simulink model "analog_digital_comp"  (R2018a)
settings: Solver=VariableStepAuto  StartTime=0.0  StopTime=5  RelTol=1e-3
values from neighbouring files (symbols this model uses):
  Fs = 2*f    (= 88200)    [Project_Script.m]
libraries: dspvision x4, commchan3 x2, commutil2 x2, dspquant2 x2, dsparch4 x1, dspsigattribs x1, dspstat3 x1
settings Model: Creator=Mehdi Raza Khorasani  LastModifiedBy=Ali
settings DataIOCC: ReturnWorkspaceOutputs=on
settings SFSimCC: SimUseLocalCustomCode=on
settings RTWCC: RTWUseLocalCustomCode=on

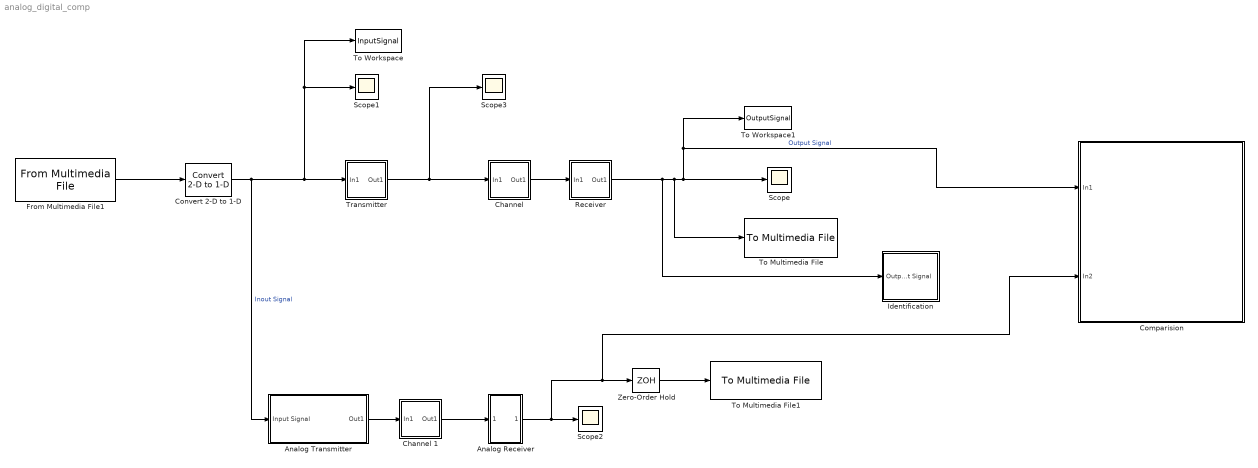
== system analog_digital_comp ==
  Analog Receiver : Subsystem
  Analog Transmitter : Subsystem
  "Channel " : Subsystem
  Channel 1 : Subsystem
  Comparision : Subsystem
  Convert 2-D to 1-D : dspsigattribs/Convert 2-D to 1-D
      settings: SourceProductBaseCode=DS
  From Multimedia File1 : dspvision/From Multimedia File  inputFilename=E:\One Drive\OneDrive - Habib University\University\6th Semester\Analog and Digital Communications\Lab\Project\mehdi_mono.mp3  loop=on  numPlays=inf  outputStreams=Audio only  videoDataType=single  audioDataType=double  inheritSampleTime=on  userDefinedSampleTime=1/30  noAudioOutput=off  isIntensityVideo=off  fourcc=RGB  colorVideoFormat=Separate color signals  outputEOF=off  dataOrg=Column-major  audioFrameSize=1  computeAudioFrameSize=off  outSamplingMode=Sample based
  Identification : Subsystem
  Receiver : Subsystem
  Scope{,1..3} (4 alike) : Scope
  To Multimedia File : dspvision/To Multimedia File  outputFilename=E:\One Drive\OneDrive - Habib University\University\6th Semester\Analog and Digital Communications\Lab\Project\output.wav  streamSelection=Audio only  videoCompressor=None (uncompressed)  audioCompressor=None (uncompressed)  imagePorts=Separate color signals  fileType=WAV  audioDatatype=16-bit integer  fourcc=RGB  videoQuality=75  mj2000CompFactor=10
  To Multimedia File1 : dspvision/To Multimedia File  outputFilename=E:\One Drive\OneDrive - Habib University\University\6th Semester\Analog and Digital Communications\Lab\Project\output_analog.wav  streamSelection=Audio only  videoCompressor=None (uncompressed)  audioCompressor=None (uncompressed)  imagePorts=Separate color signals  fileType=WAV  audioDatatype=16-bit integer  fourcc=RGB  videoQuality=75  mj2000CompFactor=10
  To Workspace : ToWorkspace  VariableName=InputSignal  SampleTime=-1
  To Workspace1 : ToWorkspace  VariableName=OutputSignal  SampleTime=-1
  Transmitter : Subsystem
  Zero-Order Hold : ZeroOrderHold  SampleTime=1/Fs
  wires:
  "Channel "/1(Out1) -> Receiver/1(In1)
  Transmitter/1(Out1) -> Scope3/1, "Channel "/1(In1)
  Receiver/1(Out1) -> Identification/1(Output Signal), To Multimedia File/1, To Workspace1/1, Comparision/1(In1), Scope/1  "Output Signal"
  From Multimedia File1/1 -> Convert 2-D to 1-D/1
  Convert 2-D to 1-D/1 -> Scope1/1, To Workspace/1, Transmitter/1(In1), Analog Transmitter/1(Input Signal)  "Inout Signal"
  Analog Transmitter/1(Out1) -> Channel 1/1(In1)
  Analog Receiver/1(Out1) -> Zero-Order Hold/1, Comparision/2(In2), Scope2/1
  Channel 1/1(Out1) -> Analog Receiver/1(In1)
  Zero-Order Hold/1 -> To Multimedia File1/1

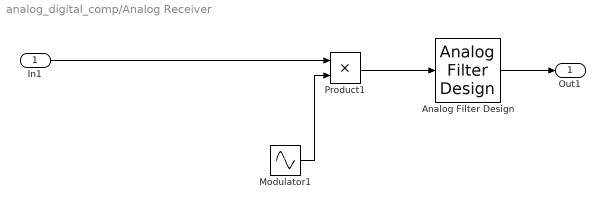
== system analog_digital_comp/Analog Receiver ==
  In1 : Inport
  Analog Filter Design : dsparch4/Analog Filter Design  method=Butterworth  filttype=Lowpass  N=8  Wlo=2*pi*15*10^3  Whi=80  Rp=2  Rs=40
  Modulator1 : Sin  Frequency=50*10^3  SampleTime=0
  Product1 : Product
  Out1 : Outport  VectorParamsAs1DForOutWhenUnconnected=on
  wires:
  Modulator1/1 -> Product1/2
  In1/1 -> Product1/1
  Analog Filter Design/1 -> Out1/1
  Product1/1 -> Analog Filter Design/1

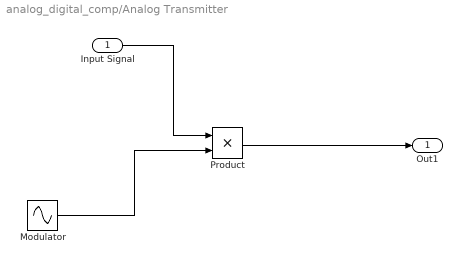
== system analog_digital_comp/Analog Transmitter ==
  Input Signal : Inport
  Modulator : Sin  Frequency=50*10^3  SampleTime=0
  Product : Product
  Out1 : Outport  VectorParamsAs1DForOutWhenUnconnected=on
  wires:
  Input Signal/1 -> Product/1
  Modulator/1 -> Product/2
  Product/1 -> Out1/1

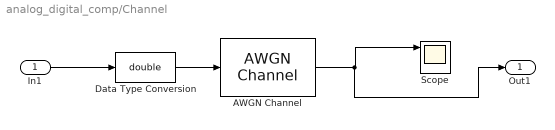
== system analog_digital_comp/Channel  ==
  In1 : Inport
  AWGN Channel : commchan3/AWGN Channel  InputProcessing=Columns as channels (frame based)  seed=67  noiseMode="Signal to noise ratio  (SNR)"  EbNodB=10  EsNodB=10  SNRdB=100  bitsPerSym=8  Ps=1  Tsym=1/Fs  variance=1
  Data Type Conversion : DataTypeConversion  OutDataTypeStr=double
  Scope : Scope  NumInputPorts=3
  Out1 : Outport  VectorParamsAs1DForOutWhenUnconnected=on
  wires:
  In1/1 -> Data Type Conversion/1
  Data Type Conversion/1 -> AWGN Channel/1
  AWGN Channel/1 -> Out1/1, Scope/1

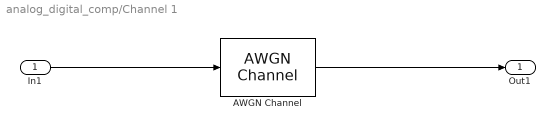
== system analog_digital_comp/Channel 1 ==
  In1 : Inport
  AWGN Channel : commchan3/AWGN Channel  InputProcessing=Columns as channels (frame based)  seed=67  noiseMode="Signal to noise ratio  (SNR)"  EbNodB=10  EsNodB=10  SNRdB=100  bitsPerSym=8  Ps=1  Tsym=1/Fs  variance=1
  Out1 : Outport  VectorParamsAs1DForOutWhenUnconnected=on
  wires:
  AWGN Channel/1 -> Out1/1
  In1/1 -> AWGN Channel/1

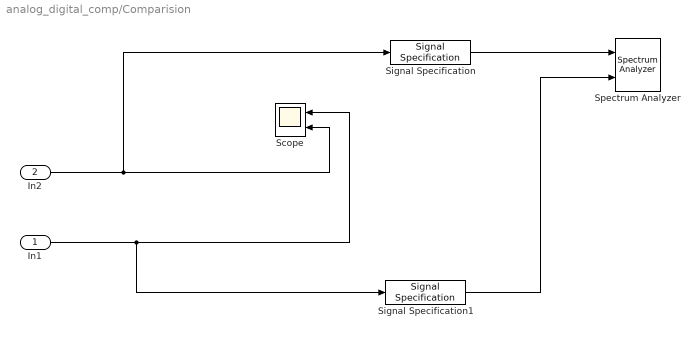
== system analog_digital_comp/Comparision ==
  In1 : Inport
  In2 : Inport  Port=2
  Scope : Scope  NumInputPorts=2
  Signal Specification : SignalSpecification  SampleTime=1/Fs
  Signal Specification1 : SignalSpecification  SampleTime=1/Fs
  Spectrum Analyzer : SpectrumAnalyzer  NumInputPorts=2
  wires:
  In1/1 -> Signal Specification1/1, Scope/1
  In2/1 -> Signal Specification/1, Scope/2
  Signal Specification/1 -> Spectrum Analyzer/1
  Signal Specification1/1 -> Spectrum Analyzer/2

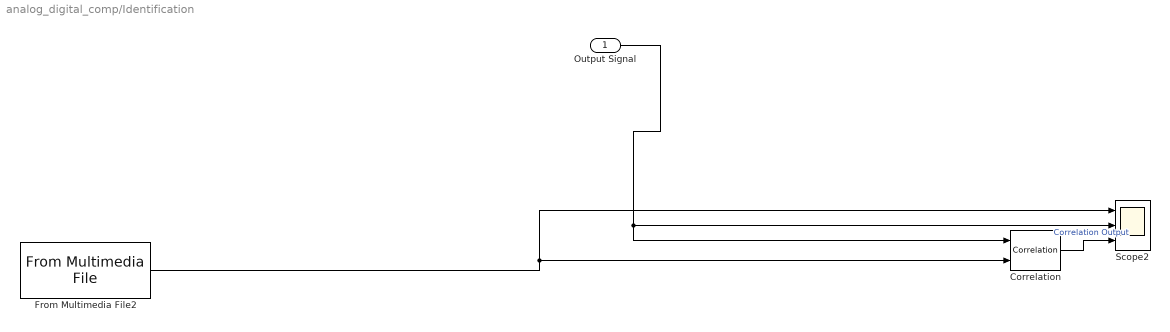
== system analog_digital_comp/Identification ==
  Output Signal : Inport
  Correlation : dspstat3/Correlation  domain=Time  roundingMode=Floor  overflowMode=off  outputDataTypeStr=Inherit: Same as accumulator  outputMin=[]  outputMax=[]  outputLastDataTypeStr=Inherit: Same as accumulator
      settings: SourceProductBaseCode=DS
  From Multimedia File2 : dspvision/From Multimedia File  inputFilename=speech_dft.mp3  loop=on  numPlays=inf  outputStreams=Audio only  videoDataType=single  audioDataType=double  inheritSampleTime=on  userDefinedSampleTime=1/30  noAudioOutput=off  isIntensityVideo=off  fourcc=RGB  colorVideoFormat=Separate color signals  outputEOF=off  dataOrg=Column-major  audioFrameSize=1  computeAudioFrameSize=off  outSamplingMode=Sample based
  Scope2 : Scope  NumInputPorts=3
  wires:
  Output Signal/1 -> Scope2/2, Correlation/1
  From Multimedia File2/1 -> Scope2/1, Correlation/2
  Correlation/1 -> Scope2/3  "Correlation Output"

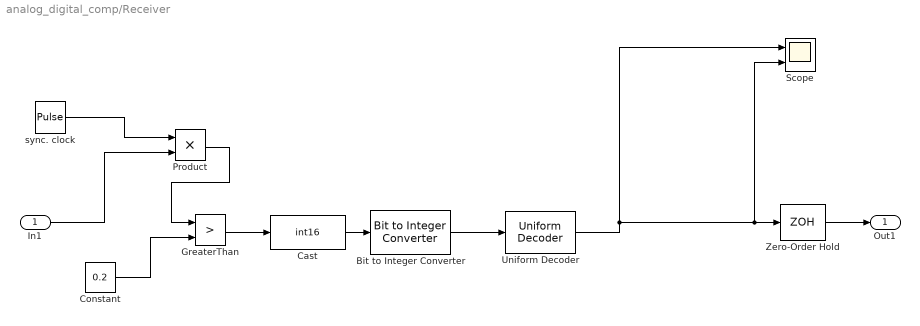
== system analog_digital_comp/Receiver ==
  In1 : Inport
  Bit to Integer Converter : commutil2/Bit to Integer Converter  nbits=bits  bitOrder=MSB first  signedOutputValues=Signed  outDtype=Inherit via internal rule  outDtypeSigned=Inherit via internal rule
  Cast : DataTypeConversion  OutDataTypeStr=int16
  Constant : Constant  Value=0.2
  GreaterThan : RelationalOperator  Operator=>  OutDataTypeStr=boolean  RndMeth=Simplest
  Product : Product
  Scope : Scope  NumInputPorts=2
  Uniform Decoder : dspquant2/Uniform Decoder  peak=5  bits=bits  overflowMode=Saturate  otype=Double
      settings: SourceProductBaseCode=DS
  Zero-Order Hold : ZeroOrderHold  SampleTime=-1
  "sync. clock " : DiscretePulseGenerator  PulseType=Time based  Period=1/Fs  PulseWidth=50
  Out1 : Outport  VectorParamsAs1DForOutWhenUnconnected=on
  wires:
  Uniform Decoder/1 -> Zero-Order Hold/1, Scope/2, Scope/1
  Bit to Integer Converter/1 -> Uniform Decoder/1
  Zero-Order Hold/1 -> Out1/1
  In1/1 -> Product/2
  Constant/1 -> GreaterThan/2
  GreaterThan/1 -> Cast/1
  Cast/1 -> Bit to Integer Converter/1
  "sync. clock "/1 -> Product/1
  Product/1 -> GreaterThan/1

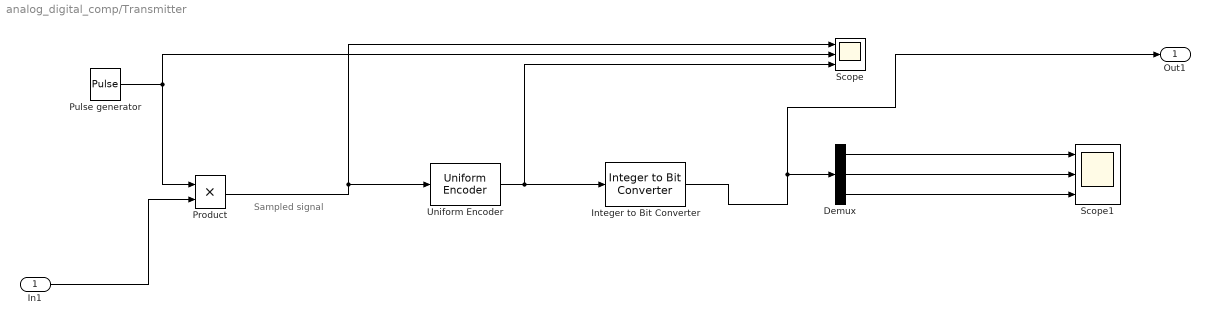
== system analog_digital_comp/Transmitter ==
  note: Sampled signal
  In1 : Inport
  Demux : Demux  Outputs=3
  Integer to Bit Converter : commutil2/Integer to Bit Converter  nbits=bits  signedInputValues=Signed  bitOrder=MSB first  outDtype=Inherit via internal rule
  Product : Product
  Pulse generator : DiscretePulseGenerator  PulseType=Time based  Period=1/Fs  PulseWidth=50
  Scope : Scope  NumInputPorts=3
  Scope1 : Scope  NumInputPorts=3
  Uniform Encoder : dspquant2/Uniform Encoder  peak=5  bits=bits  otype=Signed integer
  Out1 : Outport  VectorParamsAs1DForOutWhenUnconnected=on
  wires:
  Product/1 -> Uniform Encoder/1, Scope/1
  Demux/3 -> Scope1/3
  Uniform Encoder/1 -> Integer to Bit Converter/1, Scope/3
  Pulse generator/1 -> Product/1, Scope/2
  Demux/1 -> Scope1/1
  Demux/2 -> Scope1/2
  In1/1 -> Product/2
  Integer to Bit Converter/1 -> Out1/1, Demux/1
